simulink model "odeOrder1"  (R2021b)
settings: Solver=VariableStepAuto  StartTime=0.0  StopTime=10.0  RelTol=1e-3
settings Model: Creator=ziyutian  LastModifiedBy=ziyutian

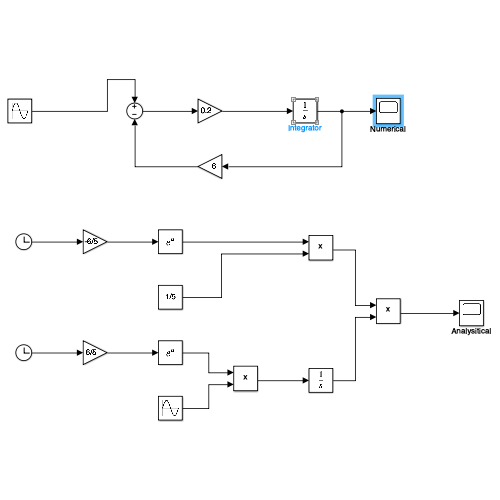
[thumbnail: Simulink's stored preview of the top-level diagram]
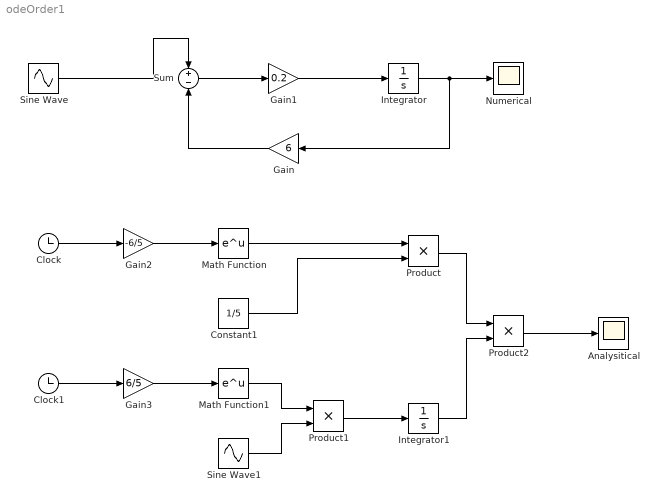
== system odeOrder1 ==
  Analysitical : Scope
  Clock : Clock
  Clock1 : Clock
  Constant1 : Constant  Value=1/5
  Gain : Gain  Gain=6
  Gain1 : Gain  Gain=0.2
  Gain2 : Gain  Gain=-6/5
  Gain3 : Gain  Gain=6/5
  Integrator : Integrator  InitialCondition=1
  Integrator1 : Integrator  InitialCondition=1
  Math Function : Math  SaturateOnIntegerOverflow=on
  Math Function1 : Math  SaturateOnIntegerOverflow=on
  Numerical : Scope
  Product : Product
  Product1 : Product
  Product2 : Product
  Sine Wave : Sin  Frequency=50  SampleTime=0
  Sine Wave1 : Sin  Frequency=50  SampleTime=0
  Sum : Sum  Inputs=+-
  wires:
  Sum/1 -> Gain1/1
  Gain1/1 -> Integrator/1
  Integrator/1 -> Gain/1, Numerical/1
  Gain/1 -> Sum/2
  Sine Wave/1 -> Sum/1
  Clock/1 -> Gain2/1
  Gain2/1 -> Math Function/1
  Math Function/1 -> Product/1
  Constant1/1 -> Product/2
  Clock1/1 -> Gain3/1
  Gain3/1 -> Math Function1/1
  Math Function1/1 -> Product1/1
  Sine Wave1/1 -> Product1/2
  Product1/1 -> Integrator1/1
  Product/1 -> Product2/1
  Integrator1/1 -> Product2/2
  Product2/1 -> Analysitical/1
